simulink model "punto1a"  (Simulink 5.0)
settings: Solver=ode45  StartTime=0.0  StopTime=20  RelTol=1e-3
settings Model: LastModifiedBy=Juan

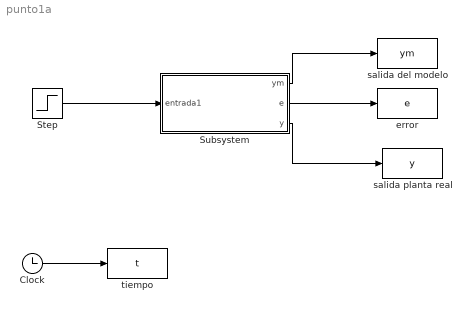
== system punto1a ==
  Clock : Clock
      settings: Decimation=10
  Step : Step  SampleTime=0
  Subsystem : Subsystem  mask{am=2, bm=2, a=1, b=1, kp=1, km=2, g=10, titainicial=0}
      mask prompts: am "a del modelo (am)"; bm "b del modelo (bm)"; a "a de la planta real (a)"; b "b de la planta real (b)"; kp "ganancia de la planta real (kp)"; km "ganancia del modelo (km)"; g "gama"; titainicial "valor inicial de tita"
      mask Display: disp('Sistema')
  error : ToWorkspace  VariableName=e  SampleTime=-1  SaveFormat=Array
  salida del modelo : ToWorkspace  VariableName=ym  SampleTime=-1  SaveFormat=Array
  salida planta real : ToWorkspace  VariableName=y  SampleTime=-1  SaveFormat=Array
  tiempo : ToWorkspace  VariableName=t  SampleTime=-1  SaveFormat=Array
  wires:
  Clock/1 -> tiempo/1
  Subsystem/1(ym) -> salida del modelo/1
  Step/1 -> Subsystem/1(entrada1)
  Subsystem/2(e) -> error/1
  Subsystem/3(y) -> salida planta real/1

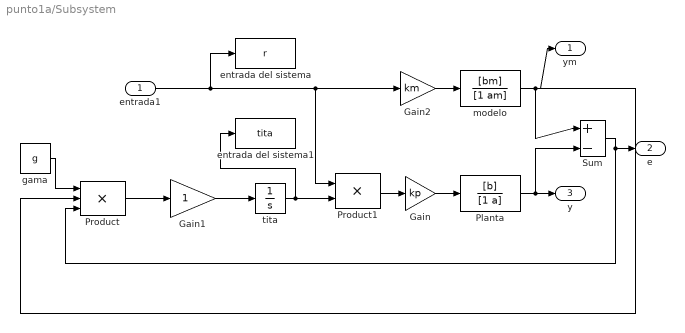
== system punto1a/Subsystem ==
  entrada1 : Inport
  Gain : Gain  Gain=kp  SaturateOnIntegerOverflow=on
  Gain1 : Gain  SaturateOnIntegerOverflow=on
  Gain2 : Gain  Gain=km  SaturateOnIntegerOverflow=on
  Planta : TransferFcn  Numerator=[b]  Denominator=[1 a]
  Product : Product  Inputs=3  SaturateOnIntegerOverflow=on
  Product1 : Product  SaturateOnIntegerOverflow=on
  Sum : Sum  Inputs=|+-  SaturateOnIntegerOverflow=on
  entrada del sistema : ToWorkspace  VariableName=r  SampleTime=-1  SaveFormat=Array
  entrada del sistema1 : ToWorkspace  VariableName=tita  SampleTime=-1  SaveFormat=Array
  gama : Constant  Value=g
  modelo : TransferFcn  Numerator=[bm]  Denominator=[1 am]
  tita : Integrator  InitialCondition=titainicial
  ym : Outport
  e : Outport  Port=2
  y : Outport  Port=3
  wires:
  Product/1 -> Gain1/1
  modelo/1 -> Sum/1, Product/2, ym/1
  Planta/1 -> Sum/2, y/1
  Product1/1 -> Gain/1
  tita/1 -> Product1/2, entrada del sistema1/1
  Gain1/1 -> tita/1
  Sum/1 -> Product/3, e/1
  gama/1 -> Product/1
  Gain2/1 -> modelo/1
  Gain/1 -> Planta/1
  entrada1/1 -> entrada del sistema/1, Product1/1, Gain2/1
